simulink model "System_parte"  (Simulink 7.2)
settings: Solver=ode45  StartTime=0.0  StopTime=2000  RelTol=1e-3
settings Model: Creator=Ehsan  LastModifiedBy=Ehsan

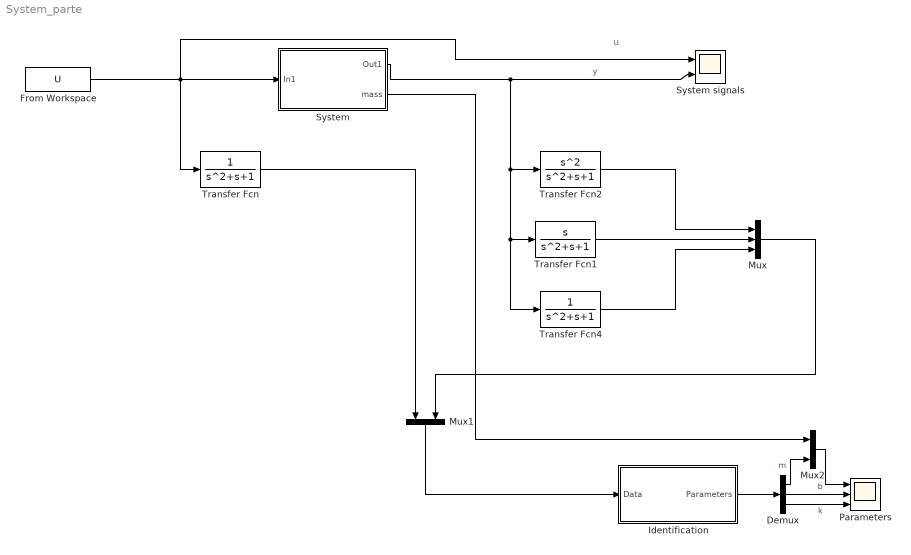
== system System_parte ==
  note: u
  Demux : Demux  Outputs=3
  From Workspace : FromWorkspace  VariableName=U  SampleTime=0
  Identification : Subsystem
  Mux : Mux  Inputs=3
  Mux1 : Mux  Orientation=down  Inputs=2
  Mux2 : Mux  Inputs=2
  Parameters : Scope  NumInputPorts=3
      settings: TimeRange=2000  YMin=-50~-20~-10  YMax=50~10~20
  System : Subsystem  InitFcn=|
      | t = 1:1:2000;                                
      | u = idinput([2000 1],'prbs',[0 2/2/pi],[0 1])
      | U = [t' , u]
  System signals : Scope  NumInputPorts=2
      settings: TimeRange=50  YMin=-5~-5  YMax=5~5
  Transfer Fcn : TransferFcn  Denominator=[1 1 1]
  Transfer Fcn1 : TransferFcn  Numerator=[1 0]  Denominator=[1 1 1]
  Transfer Fcn2 : TransferFcn  Numerator=[1 0 0]  Denominator=[1 1 1]
  Transfer Fcn4 : TransferFcn  Denominator=[1 1 1]
  wires:
  System/1(Out1) -> Transfer Fcn1/1, Transfer Fcn4/1, Transfer Fcn2/1, System signals/2  "y"
  From Workspace/1 -> Transfer Fcn/1, System signals/1, System/1(In1)
  Transfer Fcn2/1 -> Mux/1
  Transfer Fcn1/1 -> Mux/2
  Transfer Fcn4/1 -> Mux/3
  Transfer Fcn/1 -> Mux1/1
  Mux/1 -> Mux1/2
  Mux1/1 -> Identification/1(Data)
  Identification/1(Parameters) -> Demux/1
  Demux/2 -> Parameters/2  "b"
  Demux/3 -> Parameters/3  "k"
  System/2(mass) -> Mux2/1
  Demux/1 -> Mux2/2  "m"
  Mux2/1 -> Parameters/1

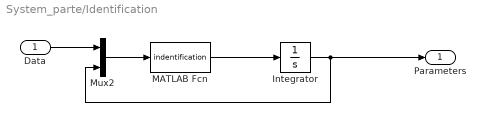
== system System_parte/Identification ==
  Data : Inport  OutDataType=sfix(16)  OutScaling=2^0
  Integrator : Integrator  InitialCondition=[10;0.05;3]
  MATLAB Fcn : MATLABFcn  MATLABFcn=indentification  OutputDimensions=3
  Mux2 : Mux  Inputs=2
  Parameters : Outport  OutDataType=sfix(16)  OutScaling=2^0
  wires:
  MATLAB Fcn/1 -> Integrator/1
  Mux2/1 -> MATLAB Fcn/1
  Data/1 -> Mux2/1
  Integrator/1 -> Mux2/2, Parameters/1

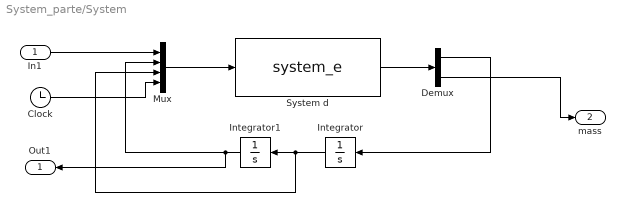
== system System_parte/System ==
  In1 : Inport  OutDataType=sfix(16)  OutScaling=2^0
  Clock : Clock
      settings: Decimation=10
  Demux : Demux  Outputs=2
  Integrator : Integrator  Orientation=left
  Integrator1 : Integrator  Orientation=left  InitialCondition=1  ContinuousStateAttributes='position'
  Mux : Mux
  System d : MATLABFcn  MATLABFcn=system_e  OutputDimensions=2
  Out1 : Outport  Orientation=left  OutDataType=sfix(16)  OutScaling=2^0
  mass : Outport  Port=2  OutDataType=sfix(16)  OutScaling=2^0
  wires:
  Mux/1 -> System d/1
  In1/1 -> Mux/1
  Integrator1/1 -> Out1/1, Mux/2
  Integrator/1 -> Mux/3, Integrator1/1
  Clock/1 -> Mux/4
  System d/1 -> Demux/1
  Demux/1 -> Integrator/1
  Demux/2 -> mass/1
